simulink model "Conor_RM3"  (R2017a)
settings: Solver=VariableStepAuto  StartTime=0.0  StopTime=10.0  RelTol=1e-3
undefined symbols (not defined in the file or in its folder): body, constraint, pto
libraries: WECSim_Lib x5
settings Model: Creator=Conor  LastModifiedBy=Conor

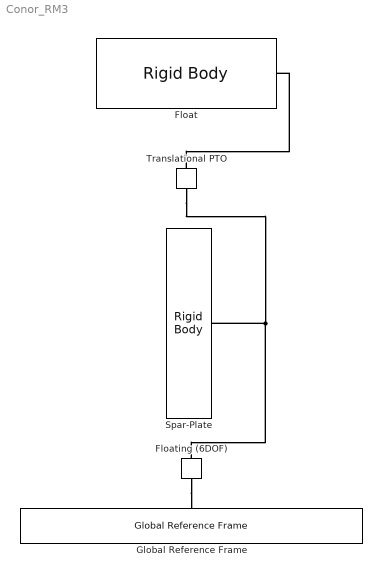
== system Conor_RM3 ==
  Float : WECSim_Lib/Body Elements/Rigid Body  body=body(1)
      settings: AttributesFormatString=%<body>  SourceProductName=WEC-Sim
  Floating (6DOF) : WECSim_Lib/Constraints/Floating (6DOF)  constraint=constraint(1)
      settings: AttributesFormatString=%<constraint>  SourceProductName=WEC-Sim
  Global Reference Frame : WECSim_Lib/Frames/Global Reference Frame  waves=noWave  simu=simu
      settings: SourceProductName=WEC-Sim
  Spar-Plate : WECSim_Lib/Body Elements/Rigid Body  body=body (2)
      settings: AttributesFormatString=%<body>  SourceProductName=WEC-Sim
  Translational PTO : WECSim_Lib/PTOs/Translational PTO  pto=pto(1)
      settings: AttributesFormatString=%<pto>  SourceProductName=WEC-Sim
  connections:
  Floating (6DOF)/RConn1 -- Global Reference Frame/RConn1
  Translational PTO/RConn1 -- Float/RConn1
  Translational PTO/LConn1 -- Floating (6DOF)/LConn1 -- Spar-Plate/RConn1
